simulink model "sm_parts_test_tube_circ"  (R2026a)
settings: Solver=VariableStepAuto  EnableMultiTasking=on
model workspace (MATLAB code in the model file):
  | circ_or = 0.3;
  | circ_ir = 0.2;
  | circ_a1 = 10;
  | circ_a2 = 85;
  | circ_arc_rad = 0.25;
  | circ_arc = 270/2;
  | circ_density = 7000;
  | circ_color = [0 0.4 0.6];
  | circ_opc = 1;
  | circ_len = 0.3;
undefined symbols (not defined in the file): X, Y, Z
libraries: Multibody_Parts_Lib x16, sm_lib x7, nesl_utility x1
CloseFcn:
  | try,close(h1_sm_parts_test_tube_circ),end
  | clear h1_sm_parts_test_tube_circ
  | try,close(h2_sm_parts_test_tube_circ),end
  | clear h2_sm_parts_test_tube_circ
  | try,close(h3_sm_parts_test_tube_circ),end
  | clear h3_sm_parts_test_tube_circ
  | try,close(h4_sm_parts_test_tube_circ),end
  | clear h4_sm_parts_test_tube_circ
Description:
  | Circular Extrusion Assembly
  | 
  | Copyright 2017-2026 The MathWorks, Inc.
settings Model: Creator=smiller  LastModifiedBy=smiller
settings DebuggingCC: PregeneratedLibrarySubsystemCodeDiagnostic=none
settings SimscapeCC: SimscapeNormalizeSystem=off  SimscapeNominalValues="[{\"value\":\"1\",\"unit\":\"A\"},{\"value\":\"1\",\"unit\":\"bar\"},{\"value\":\"1\",\"unit\":\"cm^2\"},{\"value\":\"1\",\"unit\":\"cm^3/s\"},{\"value\":\"1\",\"unit\":\"kJ/kg\"},{\"value\":\"1\",\"unit\":\"kW\"},{\"value\":\"1\",\"unit\":\"l\"},{\"value\":\"1\",\"unit\":\"N\"},{\"value\":\"1\",\"unit\":\"N*m\"},{\"value\":\"1\",\"unit\":\"V\"}]"
settings ConfigurationSet: Description=SimMechanics 2G
settings DiagnosticsConfigSet: SimMechanicsUnconnectedFramePorts=none
settings ExplorerConfigSet: InternalSimMechanicsExplorerSettings="<ExplorerConfiguration><canonicalview>planar_xy</canonicalview><AnimationSetting><BasePlaybackSpeed>1.0</BasePlaybackSpeed><PlaybackSpeedFactor>1.0</PlaybackSpeedFactor></AnimationSetting><TilePanel><TileInfo><Tiles Columns=\"2\" Count=\"2\" Rows=\"1\"><Column Left=\"2\" Weight=\"0.4992\"/><Column Left=\"305\" Weight=\"0.5008\"/><Column Left=\"608\"/><Row Top=\"2\" Weight=\"1\"/><Row Top=\"397\"/><Tile Height=\"1\" Width=\"1\" X=\"0\" Y=\"0\"/><Tile Height=\"1\" Width=\"1\" X=\"1\" Y=\"0\"/></Tiles></TileInfo><SceneInfo><SceneViewer><BGColor><R>1</R><G>1</G><B>1</B></BGColor><Camera><DoPerspective>off</DoPerspective><Position><X>-7.3519448260608824</X><Y>0.16328723738017106</Y><Z>-0.081833715246992927</Z></Position><Center><X>-1.2130681365378873</X><Y>0.16328723738017106</Y><Z>-0.081833715246992927</Z></Center><Up><X>-0</X><Y>1</Y><Z>0</Z></Up><ViewLimDist>1</ViewLimDist><YLim>1.595936423458254</YLim><XLim>1.2155577940329707</XLim></Camera></SceneViewer><SceneViewer><BGColor><R>1</R><G>1</G><B>1</B></BGColor><Camera><DoPerspective>off</DoPerspective><Position><X>-6.2113487788587838</X><Y>3.5882738337960962</Y><Z>0.46129240218885081</Z></Position><Center><X>-1.836338286043429</X><Y>2.1532273523220908</Y><Z>-2.7405911923025177</Z></Center><Up><X>0.21656061186599329</X><Y>0.96656645249549644</Y><Z>-0.13729819481150571</Z></Up><ViewLimDist>1</ViewLimDist><YLim>3.036619657283846</YLim><XLim>2.3128657493301832</XLim></Camera></SceneViewer></SceneInfo></TilePanel><MechEditorPanel><Cameras/><GfxPanelCameraMap/><VideoCreator><PlaybackSpeedRatio>1.0</PlaybackSpeedRatio><FrameRate>30</FrameRate><VideoFormat>Motion JPEG AVI</VideoFormat><FrameSize>auto</FrameSize></VideoCreator></MechEditorPanel></ExplorerConfiguration>"

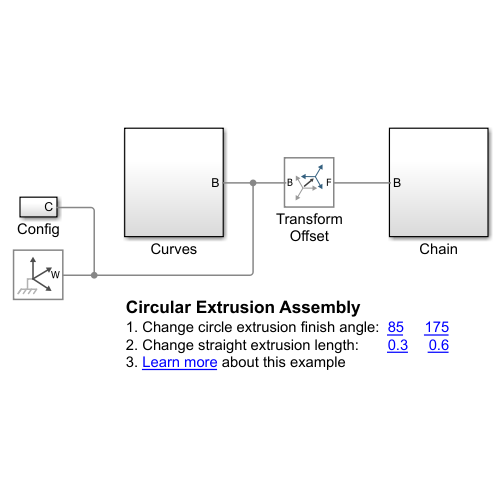
[thumbnail: Simulink's stored preview of the top-level diagram]
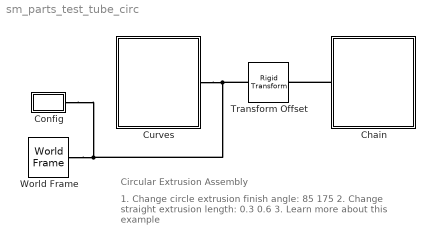
== system sm_parts_test_tube_circ ==
  note: Circular Extrusion Assembly
  note: 1. Change circle extrusion finish angle: 85 175
      | 2. Change straight extrusion length: 0.3 0.6
      | 3. Learn more about this example
  Chain : Subsystem  Tag=PublishSubsystem
  Config : Subsystem
  Curves : Subsystem  Tag=PublishSubsystem
  Transform Offset : sm_lib/Frames and Transforms/Rigid Transform  RotationMethod=None  FollAlignAxisA=+X  BaseAlignAxisA=+Y  FollAlignAxisB=+Y  BaseAlignAxisB=+Z  RotationStandardAxis=+Z  RotationAngle=0.0  RotationAngleUnits=deg  RotationArbitraryAxis=[0 0 1]  RotationSequenceAxes=FollowerAxes  RotationSequence=XYX  RotationSequenceAngles=[0 0 0]  RotationSequenceAnglesUnits=deg  RotationMatrix=[1 0 0; 0 1 0; 0 0 1]  Quaternion=[1 0 0 0]  TranslationMethod=StandardAxis  TranslationCartesianOffset=[0 0 0]  TranslationCartesianOffsetUnits=m  TranslationStandardAxis=+Z  TranslationStandardOffset=-2  TranslationStandardOffsetUnits=m  TranslationROffset=0  TranslationROffsetUnits=m  TranslationThetaOffset=0  TranslationThetaOffsetUnits=deg  TranslationZOffset=0  TranslationZOffsetUnits=m
  World Frame : sm_lib/Frames and Transforms/World Frame
  connections:
  Chain/LConn1 -- Transform Offset/RConn1
  Curves/LConn1 -- Config/LConn1 -- World Frame/RConn1 -- Transform Offset/LConn1

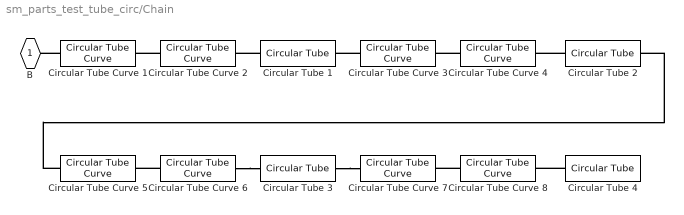
== system sm_parts_test_tube_circ/Chain ==
  Circular Tube {1..4} (4 alike) : Multibody_Parts_Lib/Extrusions/Circular Tube  circ_radout=circ_or  circ_radin=circ_ir  deg_1=circ_a1  deg_2=circ_a2  circ_len=circ_len  circ_rho=circ_density  circ_color=[0.2 0.6 0.2]  circ_opc=circ_opc
      settings: SourceProductName=Simscape Multibody Parts Library
  Circular Tube Curve 1 : Multibody_Parts_Lib/Extrusions/Circular Tube Curve  circ_radout=circ_or  circ_radin=circ_ir  deg_1=circ_a1  deg_2=circ_a2  arc_rad=1  arc_angle=circ_arc  popup_arcdir=Z  circ_rho=circ_density  circ_color=circ_color  circ_opc=circ_opc
      settings: SourceProductName=Simscape Multibody Parts Library
  Circular Tube Curve 2 : Multibody_Parts_Lib/Extrusions/Circular Tube Curve  circ_radout=circ_or  circ_radin=circ_ir  deg_1=circ_a1  deg_2=circ_a2  arc_rad=1  arc_angle=circ_arc  popup_arcdir=Z  circ_rho=circ_density  circ_color=circ_color  circ_opc=circ_opc
      settings: SourceProductName=Simscape Multibody Parts Library
  Circular Tube Curve 3 : Multibody_Parts_Lib/Extrusions/Circular Tube Curve  circ_radout=circ_or  circ_radin=circ_ir  deg_1=circ_a1  deg_2=circ_a2  arc_rad=1  arc_angle=circ_arc  popup_arcdir=Y  circ_rho=circ_density  circ_color=circ_color  circ_opc=circ_opc
      settings: SourceProductName=Simscape Multibody Parts Library
  Circular Tube Curve 4 : Multibody_Parts_Lib/Extrusions/Circular Tube Curve  circ_radout=circ_or  circ_radin=circ_ir  deg_1=circ_a1  deg_2=circ_a2  arc_rad=1  arc_angle=circ_arc  popup_arcdir=Y  circ_rho=circ_density  circ_color=circ_color  circ_opc=circ_opc
      settings: SourceProductName=Simscape Multibody Parts Library
  Circular Tube Curve 5 : Multibody_Parts_Lib/Extrusions/Circular Tube Curve  circ_radout=circ_or  circ_radin=circ_ir  deg_1=circ_a1  deg_2=circ_a2  arc_rad=1  arc_angle=-circ_arc  popup_arcdir=Z  circ_rho=circ_density  circ_color=circ_color  circ_opc=circ_opc
      settings: SourceProductName=Simscape Multibody Parts Library
  Circular Tube Curve 6 : Multibody_Parts_Lib/Extrusions/Circular Tube Curve  circ_radout=circ_or  circ_radin=circ_ir  deg_1=circ_a1  deg_2=circ_a2  arc_rad=1  arc_angle=-circ_arc  popup_arcdir=Z  circ_rho=circ_density  circ_color=circ_color  circ_opc=circ_opc
      settings: SourceProductName=Simscape Multibody Parts Library
  Circular Tube Curve 7 : Multibody_Parts_Lib/Extrusions/Circular Tube Curve  circ_radout=circ_or  circ_radin=circ_ir  deg_1=circ_a1  deg_2=circ_a2  arc_rad=1  arc_angle=-circ_arc  popup_arcdir=Y  circ_rho=circ_density  circ_color=circ_color  circ_opc=circ_opc
      settings: SourceProductName=Simscape Multibody Parts Library
  Circular Tube Curve 8 : Multibody_Parts_Lib/Extrusions/Circular Tube Curve  circ_radout=circ_or  circ_radin=circ_ir  deg_1=circ_a1  deg_2=circ_a2  arc_rad=1  arc_angle=-circ_arc  popup_arcdir=Y  circ_rho=circ_density  circ_color=circ_color  circ_opc=circ_opc
      settings: SourceProductName=Simscape Multibody Parts Library
  B : PMIOPort  Side=Left
  connections:
  Circular Tube Curve 1/LConn1 -- B/RConn1
  Circular Tube Curve 2/LConn1 -- Circular Tube Curve 1/RConn1
  Circular Tube Curve 4/LConn1 -- Circular Tube Curve 3/RConn1
  Circular Tube 1/LConn1 -- Circular Tube Curve 2/RConn1
  Circular Tube Curve 6/LConn1 -- Circular Tube Curve 5/RConn1
  Circular Tube Curve 8/LConn1 -- Circular Tube Curve 7/RConn1
  Circular Tube 2/LConn1 -- Circular Tube Curve 4/RConn1
  Circular Tube Curve 6/RConn1 -- Circular Tube 3/LConn1
  Circular Tube Curve 3/LConn1 -- Circular Tube 1/RConn1
  Circular Tube Curve 5/LConn1 -- Circular Tube 2/RConn1
  Circular Tube 3/RConn1 -- Circular Tube Curve 7/LConn1
  Circular Tube 4/LConn1 -- Circular Tube Curve 8/RConn1

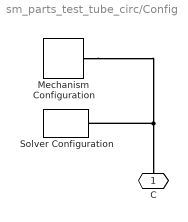
== system sm_parts_test_tube_circ/Config ==
  Mechanism Configuration : sm_lib/Utilities/Mechanism Configuration  UniformGravity=Constant  GravityVector=[0 -1 0]*9.80665  GravityVectorUnits=m/s^2  LinearizationDelta=0.001  JointModeTransitionNonlinearIterations=2
  Solver Configuration : nesl_utility/Solver Configuration  PhysicalDomain=network_engine_domain  SubClassName=solver  LeftPortType=input  RightPortType=generic  Tones=[]  Harmonics=[]  SimulateNoise=off  Profile=off  UseLocalSampling=off  EnableSwitchedLinearOptims=on  FrequencyDomain=off  UseCCode=off  RelTol=0.001  AbsTol=1e-06  MinStep=1e-09  ToWorkspace=off  RevertToSquareIcSolve=off  NumHomotopyIterations=100  PhasorMode=off  PhasorModeNumHarmonics=1  ConsistencySolver=NEWTON_FTOL  CanonicalOrdering=UNORDERED  OptimizeIntermediates=UNOPTIMIZED  IndexReductionMethod=DerivativeReplacement  DoDC=off  ResidualTolerance=1e-09  ConsistencyTolSource=GLOBAL  ConsistencyAbsTol=0.001  ConsistencyRelTol=0.001  ConsistencyTolFactor=0.001  UseLocalSolver=off  LocalSolverChoice=NE_BACKWARD_EULER_ADVANCER  ResolveIndetEquations=on  FunctionEvalNumThread=1  LocalSolverSampleTime=0.001  DoFixedCost=off  MaxNonlinIter=3  MaxModeIter=2  ComputeImpulses=off  ImpulseIterations=2  LinearAlgebra=Sparse  LinearAlgebraNumThread=0  EquationFormulation=NE_TIME_EF  DelaysMemoryBudget=1024  AutomaticFiltering=on  FilteringTimeConstant=0.001  PartitionStorageMethod=AS_NEEDED  PartitionMemoryBudget=1024  PartitionMethod=FAST  MultibodyUseLocalSolver=off  MultibodyLocalSolverChoice=ODE1  MultibodyLocalSolverSampleTime=0.001
  C : PMIOPort  Side=Left
  connections:
  Mechanism Configuration/RConn1 -- Solver Configuration/RConn1 -- C/RConn1

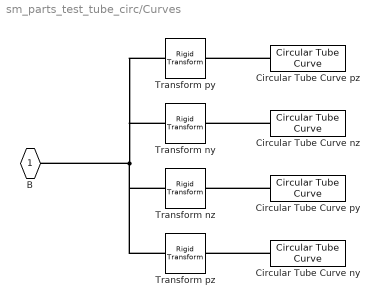
== system sm_parts_test_tube_circ/Curves ==
  Circular Tube Curve ny : Multibody_Parts_Lib/Extrusions/Circular Tube Curve  circ_radout=circ_or  circ_radin=circ_ir  deg_1=circ_a1  deg_2=circ_a2  arc_rad=1  arc_angle=-60  popup_arcdir=Y  circ_rho=circ_density  circ_color=circ_color  circ_opc=circ_opc
      settings: SourceProductName=Simscape Multibody Parts Library
  Circular Tube Curve nz : Multibody_Parts_Lib/Extrusions/Circular Tube Curve  circ_radout=circ_or  circ_radin=circ_ir  deg_1=circ_a1  deg_2=circ_a2  arc_rad=1  arc_angle=-60  popup_arcdir=Z  circ_rho=circ_density  circ_color=circ_color  circ_opc=circ_opc
      settings: SourceProductName=Simscape Multibody Parts Library
  Circular Tube Curve py : Multibody_Parts_Lib/Extrusions/Circular Tube Curve  circ_radout=circ_or  circ_radin=circ_ir  deg_1=circ_a1  deg_2=circ_a2  arc_rad=1  arc_angle=60  popup_arcdir=Y  circ_rho=circ_density  circ_color=circ_color  circ_opc=circ_opc
      settings: SourceProductName=Simscape Multibody Parts Library
  Circular Tube Curve pz : Multibody_Parts_Lib/Extrusions/Circular Tube Curve  circ_radout=circ_or  circ_radin=circ_ir  deg_1=circ_a1  deg_2=circ_a2  arc_rad=1  arc_angle=60  popup_arcdir=Z  circ_rho=circ_density  circ_color=circ_color  circ_opc=circ_opc
      settings: SourceProductName=Simscape Multibody Parts Library
  Transform ny : sm_lib/Frames and Transforms/Rigid Transform  RotationMethod=None  FollAlignAxisA=+X  BaseAlignAxisA=+Y  FollAlignAxisB=+Y  BaseAlignAxisB=+Z  RotationStandardAxis=+Z  RotationAngle=0.0  RotationAngleUnits=deg  RotationArbitraryAxis=[0 0 1]  RotationSequenceAxes=FollowerAxes  RotationSequence=XYX  RotationSequenceAngles=[0 0 0]  RotationSequenceAnglesUnits=deg  RotationMatrix=[1 0 0; 0 1 0; 0 0 1]  Quaternion=[1 0 0 0]  TranslationMethod=StandardAxis  TranslationCartesianOffset=[0 0 0]  TranslationCartesianOffsetUnits=m  TranslationStandardAxis=+Y  TranslationStandardOffset=-0.5  TranslationStandardOffsetUnits=m  TranslationROffset=0  TranslationROffsetUnits=m  TranslationThetaOffset=0  TranslationThetaOffsetUnits=deg  TranslationZOffset=0  TranslationZOffsetUnits=m
  Transform nz : sm_lib/Frames and Transforms/Rigid Transform  RotationMethod=None  FollAlignAxisA=+X  BaseAlignAxisA=+Y  FollAlignAxisB=+Y  BaseAlignAxisB=+Z  RotationStandardAxis=+Z  RotationAngle=0.0  RotationAngleUnits=deg  RotationArbitraryAxis=[0 0 1]  RotationSequenceAxes=FollowerAxes  RotationSequence=XYX  RotationSequenceAngles=[0 0 0]  RotationSequenceAnglesUnits=deg  RotationMatrix=[1 0 0; 0 1 0; 0 0 1]  Quaternion=[1 0 0 0]  TranslationMethod=StandardAxis  TranslationCartesianOffset=[0 0 0]  TranslationCartesianOffsetUnits=m  TranslationStandardAxis=+Z  TranslationStandardOffset=-0.5  TranslationStandardOffsetUnits=m  TranslationROffset=0  TranslationROffsetUnits=m  TranslationThetaOffset=0  TranslationThetaOffsetUnits=deg  TranslationZOffset=0  TranslationZOffsetUnits=m
  Transform py : sm_lib/Frames and Transforms/Rigid Transform  RotationMethod=None  FollAlignAxisA=+X  BaseAlignAxisA=+Y  FollAlignAxisB=+Y  BaseAlignAxisB=+Z  RotationStandardAxis=+Z  RotationAngle=0.0  RotationAngleUnits=deg  RotationArbitraryAxis=[0 0 1]  RotationSequenceAxes=FollowerAxes  RotationSequence=XYX  RotationSequenceAngles=[0 0 0]  RotationSequenceAnglesUnits=deg  RotationMatrix=[1 0 0; 0 1 0; 0 0 1]  Quaternion=[1 0 0 0]  TranslationMethod=StandardAxis  TranslationCartesianOffset=[0 0 0]  TranslationCartesianOffsetUnits=m  TranslationStandardAxis=+Y  TranslationStandardOffset=0.5  TranslationStandardOffsetUnits=m  TranslationROffset=0  TranslationROffsetUnits=m  TranslationThetaOffset=0  TranslationThetaOffsetUnits=deg  TranslationZOffset=0  TranslationZOffsetUnits=m
  Transform pz : sm_lib/Frames and Transforms/Rigid Transform  RotationMethod=None  FollAlignAxisA=+X  BaseAlignAxisA=+Y  FollAlignAxisB=+Y  BaseAlignAxisB=+Z  RotationStandardAxis=+Z  RotationAngle=0.0  RotationAngleUnits=deg  RotationArbitraryAxis=[0 0 1]  RotationSequenceAxes=FollowerAxes  RotationSequence=XYX  RotationSequenceAngles=[0 0 0]  RotationSequenceAnglesUnits=deg  RotationMatrix=[1 0 0; 0 1 0; 0 0 1]  Quaternion=[1 0 0 0]  TranslationMethod=StandardAxis  TranslationCartesianOffset=[0 0 0]  TranslationCartesianOffsetUnits=m  TranslationStandardAxis=+Z  TranslationStandardOffset=0.5  TranslationStandardOffsetUnits=m  TranslationROffset=0  TranslationROffsetUnits=m  TranslationThetaOffset=0  TranslationThetaOffsetUnits=deg  TranslationZOffset=0  TranslationZOffsetUnits=m
  B : PMIOPort  Side=Left
  connections:
  Transform pz/LConn1 -- Transform nz/LConn1 -- B/RConn1 -- Transform ny/LConn1 -- Transform py/LConn1
  Circular Tube Curve pz/LConn1 -- Transform py/RConn1
  Circular Tube Curve nz/LConn1 -- Transform ny/RConn1
  Circular Tube Curve py/LConn1 -- Transform nz/RConn1
  Circular Tube Curve ny/LConn1 -- Transform pz/RConn1
